simulink model "filter6"  (R2020b)
settings: Solver=VariableStepAuto  StartTime=0.0  StopTime=10.0  RelTol=1e-3
settings Model: Creator=shivanshu shukla  LastModifiedBy=shivanshu shukla

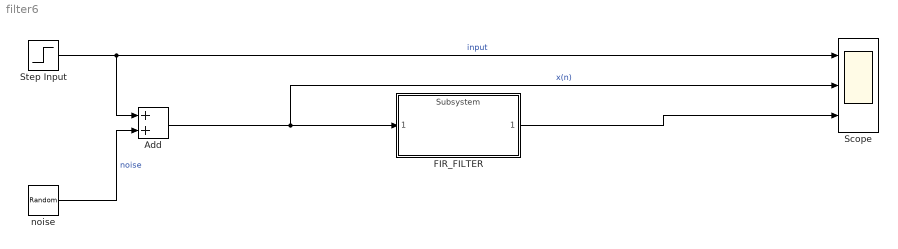
== system filter6 ==
  Add : Sum
  FIR_FILTER : ModelReference  ModelNameDialog=Subsystem  SimulationMode=Normal  ModelReferenceVersion=1.2
  Scope : Scope  NumInputPorts=3
  Step Input : Step  After=5  SampleTime=0
  noise : RandomNumber  SampleTime=0.1
  wires:
  Add/1 -> FIR_FILTER/1, Scope/2  "x(n)"
  noise/1 -> Add/2  "noise"
  Step Input/1 -> Add/1, Scope/1  "input"
  FIR_FILTER/1 -> Scope/3
